simulink model "proximity_sensor"  (R2018b)
settings: Solver=VariableStepAuto  StartTime=0.0  StopTime=11  RelTol=1e-3
libraries: simulink x1
settings Model: Creator=mikoto  LastModifiedBy=mikoto

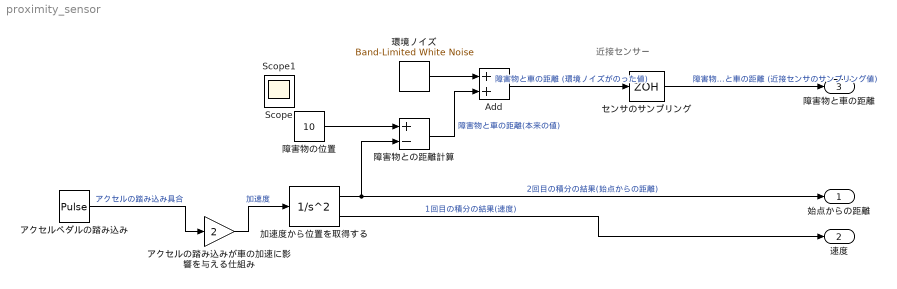
== system proximity_sensor ==
  note: 近接センサー
  Add : Sum
  アクセルの踏み込みが車の加速に影響を与える仕組み : Gain  Gain=2
  "アクセルペダルの踏み込み " : DiscretePulseGenerator  PulseType=Time based  Period=10  PulseWidth=5
  センサのサンプリング : ZeroOrderHold  SampleTime=0.1
  加速度から位置を取得する : SecondOrderIntegrator  ICX=0  UpperLimitX=10
  環境ノイズ : simulink/Sources/Band-Limited White Noise  Cov=0.001  Ts=0.1  seed=[23341]
  障害物との距離計算 : Sum  Inputs=+-
  障害物の位置 : Constant  Value=10
  始点からの距離 : Outport
  速度 : Outport  Port=2
  障害物と車の距離 : Outport  Port=3
  Scope : Scope
  Scope1 : Scope
  wires:
  "アクセルペダルの踏み込み "/1 -> アクセルの踏み込みが車の加速に影響を与える仕組み/1  "アクセルの踏み込み具合"
  アクセルの踏み込みが車の加速に影響を与える仕組み/1 -> 加速度から位置を取得する/1  "加速度"
  加速度から位置を取得する/1 -> 始点からの距離/1, 障害物との距離計算/2  "2回目の積分の結果(始点からの距離)"
  加速度から位置を取得する/2 -> 速度/1  "1回目の積分の結果(速度)"
  障害物の位置/1 -> 障害物との距離計算/1
  Add/1 -> センサのサンプリング/1  "障害物と車の距離 (環境ノイズがのった値)"
  環境ノイズ/1 -> Add/1
  障害物との距離計算/1 -> Add/2  "障害物と車の距離(本来の値)"
  センサのサンプリング/1 -> 障害物と車の距離/1  "障害物と車の距離 (近接センサのサンプリング値)"
